simulink model "BPSK_RaisedCosine_Nishat"  (R2018a)
settings: Solver=VariableStepAuto  StartTime=0.0  StopTime=inf  RelTol=1e-3
InitFcn:
  | Tb = 0.001;
  | fs = 1e4;
  | Ts = 1/fs;
  | frameSize = 1000;
libraries: commdigbbndpm3 x2, commfilt2 x2, commchan3 x1, commrandsrc3 x1, commsink2 x1, simulink x1
settings Model: SimulationMode=accelerator  Creator=prust  LastModifiedBy=n53s123
settings CodeAppCC: StateflowObjectComments=on

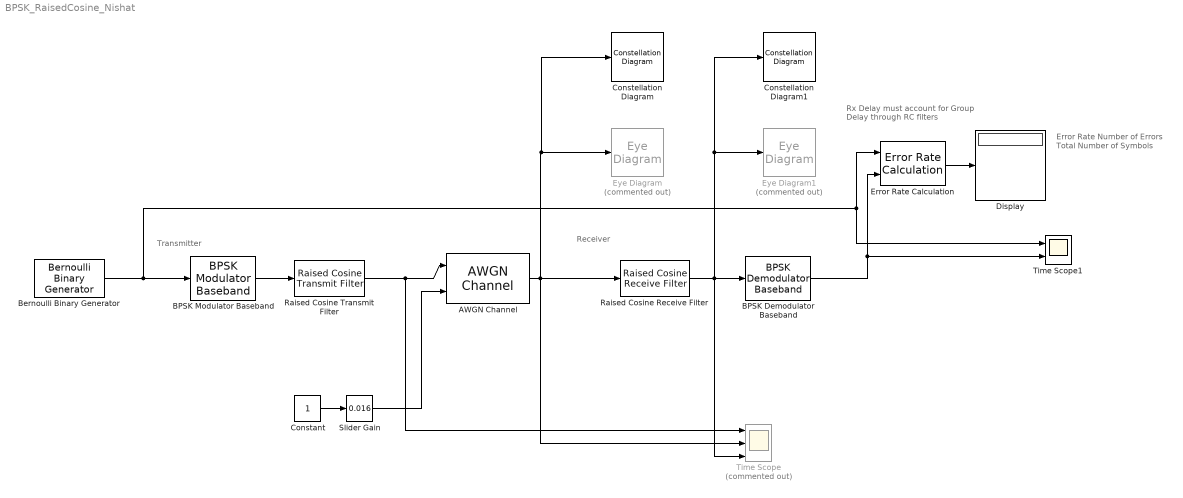
== system BPSK_RaisedCosine_Nishat ==
  note: Rx Delay must account for Group Delay through RC filters
  note: Receiver
  note: Transmitter
  note: Error Rate
      |
      | Number of Errors
      |
      | Total Number of Symbols
  AWGN Channel : commchan3/AWGN Channel  InputProcessing=Columns as channels (frame based)  seed=67  noiseMode=Variance from port  EbNodB=12  EsNodB=10  SNRdB=10  bitsPerSym=1  Ps=1  Tsym=Tb  variance=1
  BPSK Demodulator Baseband : commdigbbndpm3/BPSK Demodulator Baseband  DecType=Hard decision  VarSource=Dialog  Variance=1  Ph=0  outDtype=Inherit via internal rule  derotateFactorWordLen=16  derotateFactorDataTypeStr=Inherit: Same word length as input  derotateFactorLastDataTypeStr=Inherit: Same word length as input
  BPSK Modulator Baseband : commdigbbndpm3/BPSK Modulator Baseband  Ph=0  outDtype=double  outWordLen=16  outUDDataType=sfix(16)  outFracLenMode=Best precision  outFracLen=15  outDataTypeStr=double  outLastDataTypeStr=double
  Bernoulli Binary Generator : commrandsrc3/Bernoulli Binary Generator  ProbabilityOfZero=0.5  SeedSource=Auto  Seed=0  SampleTime=Tb  SamplesPerFrame=frameSize  OutputDataType=double  SimulateUsing=Interpreted execution
  Constant : Constant
  Constellation Diagram : ConstellationDiagram
  Constellation Diagram1 : ConstellationDiagram
  Display : Display
  Error Rate Calculation : commsink2/Error Rate Calculation  N=10  st_delay=0  cp_mode=Entire frame  subframe=[]  PMode=Port  WsName=ErrorVec  RsMode2=off  stop=off  numErr=100  maxBits=1e6
  Eye Diagram : EyeDiagram  Commented=on
  Eye Diagram1 : EyeDiagram  Commented=on
  Raised Cosine Receive Filter : commfilt2/Raised Cosine Receive Filter  filtType=Square root  R=0.2  filtSpan=10  N=Tb/Ts  downFactor=Tb/Ts  downOffset=0  filterGain=1  InputProcessing=Columns as channels (frame based)  RateOptions=Enforce single-rate processing  framing=Mute  checkCoeff=off  variableName=rcRxFilt  currentFiltSpan=10  D=(10)/2  inputOffset=0  sampMode=Mute  saveAsFlag=0  rateMode=Downsampling  checkGain=Normalized  launchFVT=on  roundingMode=Floor  overflowMode=off  coeffDataTypeStr=Inherit: Same word length as input  coeffMin=[]  coeffMax=[]  coeffLastDataTypeStr=Inherit: Same word length as input  accumDataTypeStr=Inherit: Same as product output  accumLastDataTypeStr=Inherit: Same as product output  outputDataTypeStr=Inherit: Same as accumulator  outputMin=[]  outputMax=[]  outputLastDataTypeStr=Inherit: Same as accumulator
  Raised Cosine Transmit Filter : commfilt2/Raised Cosine Transmit Filter  filtType=Square root  R=0.2  filtSpan=10  N=Tb/Ts  filterGain=1  InputProcessing=Columns as channels (frame based)  RateOptions=Enforce single-rate processing  framing=Mute  checkCoeff=off  variableName=rcTxFilt  checkGain=Normalized  sampMode=Mute  saveAsFlag=0  currentFiltSpan=10  D=(10)/2  launchFVT=on  roundingMode=Floor  overflowMode=off  coeffDataTypeStr=Inherit: Same word length as input  coeffMin=[]  coeffMax=[]  coeffLastDataTypeStr=Inherit: Same word length as input  outputDataTypeStr=Inherit: Same as accumulator  outputMin=[]  outputMax=[]  outputLastDataTypeStr=Inherit: Same as accumulator
  Slider Gain : simulink/Math Operations/Slider Gain  gain=0.016  low=0  high=.2
  Time Scope : Scope  Commented=on  NumInputPorts=3
  Time Scope1 : Scope  NumInputPorts=2
  wires:
  Bernoulli Binary Generator/1 -> BPSK Modulator Baseband/1, Time Scope1/1, Error Rate Calculation/1
  AWGN Channel/1 -> Raised Cosine Receive Filter/1, Constellation Diagram/1, Eye Diagram/1, Time Scope/2
  BPSK Demodulator Baseband/1 -> Time Scope1/2, Error Rate Calculation/2
  Error Rate Calculation/1 -> Display/1
  Raised Cosine Transmit Filter/1 -> AWGN Channel/1, Time Scope/1
  BPSK Modulator Baseband/1 -> Raised Cosine Transmit Filter/1
  Raised Cosine Receive Filter/1 -> BPSK Demodulator Baseband/1, Constellation Diagram1/1, Eye Diagram1/1, Time Scope/3
  Constant/1 -> Slider Gain/1
  Slider Gain/1 -> AWGN Channel/2
